simulink model "MyTwoTankSystem_SteadyState"  (R2021b)
settings: Solver=ode4  StartTime=0.0  StopTime=SIM_TIME  FixedStep=STEP_SIZE  RelTol=1e-3  EnableMultiTasking=on
undefined symbols (not defined in the file): At, C0, Dv, ka, kh, kt, u10, u20, v10, v20, v30, x0
settings Model: Creator=tanzc  LastModifiedBy=tanzc
settings DataIOCC: InitialState=x0  LimitDataPoints=on  SaveFinalState=on  SaveFormat=Array  ReturnWorkspaceOutputs=off

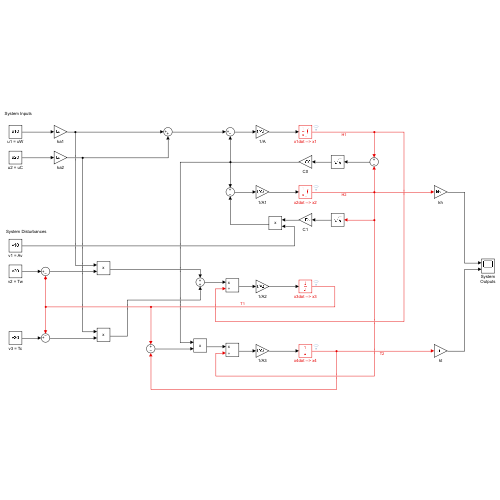
[thumbnail: Simulink's stored preview of the top-level diagram]
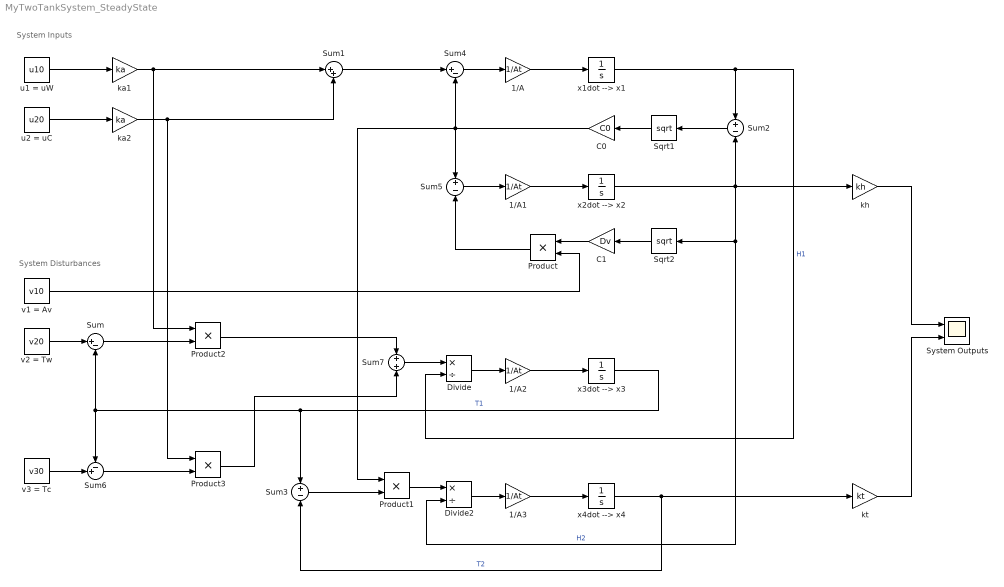
== system MyTwoTankSystem_SteadyState ==
  note: System Disturbances
  note: System Inputs
  1/A{,1..3} (4 alike) : Gain  Gain=1/At
  C0 : Gain  Gain=C0
  C1 : Gain  Gain=Dv
  Divide : Product  Inputs=*/
  Divide2 : Product  Inputs=*/
  Product{,1..3} (4 alike) : Product
  Sqrt1 : Sqrt  SaturateOnIntegerOverflow=on
  Sqrt2 : Sqrt  SaturateOnIntegerOverflow=on
  Sum : Sum  Inputs=|+-
  Sum1 : Sum  Inputs=|++
  Sum2 : Sum  Inputs=+-
  Sum3 : Sum  Inputs=+-
  Sum4 : Sum  Inputs=|+-
  Sum5 : Sum  Inputs=+-
  Sum6 : Sum  Inputs=-+|
  Sum7 : Sum
  System Outputs : Scope  NumInputPorts=2
  ka1 : Gain  Gain=ka
  ka2 : Gain  Gain=ka
  kh : Gain  Gain=kh
  kt : Gain  Gain=kt
  u1 = uW : Constant  Value=u10
  u2 = uC : Constant  Value=u20
  v1 = Av : Constant  Value=v10
  v2 = Tw : Constant  Value=v20
  v3 = Tc : Constant  Value=v30
  x1dot --> x1 : Integrator  Priority=1  InitialCondition=x0(1)  LimitOutput=on  LowerSaturationLimit=0
  x2dot --> x2 : Integrator  Priority=2  InitialCondition=x0(2)  LimitOutput=on  LowerSaturationLimit=0
  x3dot --> x3 : Integrator  Priority=3  InitialCondition=x0(3)
  x4dot --> x4 : Integrator  Priority=4  InitialCondition=x0(4)
  wires:
  Sum4/1 -> 1/A/1
  x1dot --> x1/1 -> Sum2/1, Divide/2  "H1"
  u2 = uC/1 -> ka2/1
  Sum5/1 -> 1/A1/1
  Sum7/1 -> Divide/1
  Sum2/1 -> Sqrt1/1
  u1 = uW/1 -> ka1/1
  v3 = Tc/1 -> Sum6/2
  kt/1 -> System Outputs/2
  1/A/1 -> x1dot --> x1/1
  v1 = Av/1 -> Product/2
  v2 = Tw/1 -> Sum/1
  x2dot --> x2/1 -> kh/1, Divide2/2, Sqrt2/1, Sum2/2  "H2"
  kh/1 -> System Outputs/1
  ka2/1 -> Product3/1, Sum1/2
  Sum1/1 -> Sum4/1
  ka1/1 -> Product2/1, Sum1/1
  Sum6/1 -> Product3/2
  1/A2/1 -> x3dot --> x3/1
  x4dot --> x4/1 -> kt/1, Sum3/2  "T2"
  Product/1 -> Sum5/2
  Sum3/1 -> Product1/2
  Divide2/1 -> 1/A3/1
  Sqrt2/1 -> C1/1
  Sum/1 -> Product2/2
  1/A3/1 -> x4dot --> x4/1
  Divide/1 -> 1/A2/1
  Product3/1 -> Sum7/2
  C0/1 -> Sum4/2, Product1/1, Sum5/1
  x3dot --> x3/1 -> Sum3/1, Sum6/1, Sum/2  "T1"
  Product2/1 -> Sum7/1
  Product1/1 -> Divide2/1
  Sqrt1/1 -> C0/1
  1/A1/1 -> x2dot --> x2/1
  C1/1 -> Product/1
